simulink model "DCDC3_OL"  (R2024a)
settings: Solver=ode14x  StartTime=0.0  StopTime=0.1  FixedStep=Tstep  RelTol=1e-3
values from neighbouring files (symbols this model uses):
  D_3 = (1 - (VinNom-VdropL)/VoutNom) + deadtimesw/Tsw    (= 0.428146333333)    [DCDC_param.m]
  deadtimesw = 2.8e-6    (= 2.8e-06)    [DCDC_param.m]
  IoutNom = PCN/VoutNom    (= 1.5)    [DCDC_param.m]
  Rload = VoutNom/IoutNom    (= 33.3333333333)    [DCDC_param.m]
  RserL = 8.78e-3    (= 0.00878)    [DCDC_param.m]
  Tsw = 1/fsw    (= 0.0001)    [DCDC_param.m]    (also in adcpwm_setup.m)
  VinNom = 30    [DCDC_param.m]
  VoutNom = 50    [DCDC_param.m]
undefined symbols (not defined in the file or in its folder): den_aaf, num_aaf, Tstep
libraries: fl_lib x18, nesl_utility x17, simulink x6, spsTriangleGeneratorLib x6, ee_lib x6
settings Model: Creator=nicholas  LastModifiedBy=nicholas
settings RTWCC: GPUComputeCapability=3.5

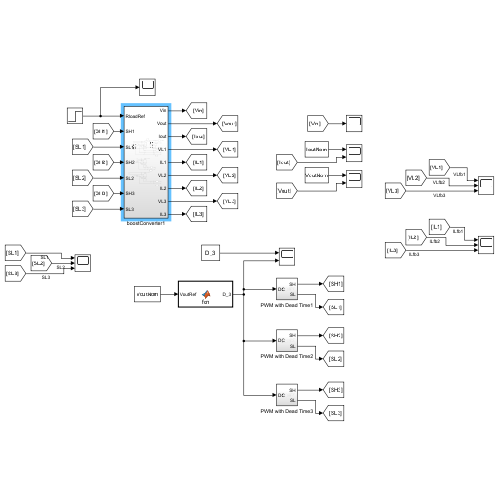
[thumbnail: Simulink's stored preview of the top-level diagram]
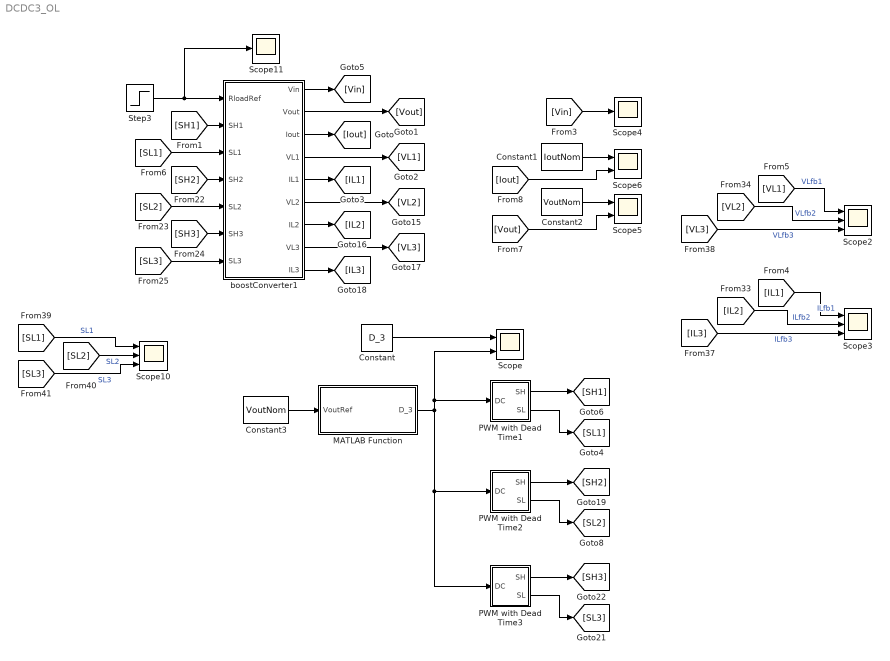
== system DCDC3_OL ==
  Constant : Constant  Value=D_3
  Constant1 : Constant  Value=IoutNom
  Constant2 : Constant  Value=VoutNom
  Constant3 : Constant  Value=VoutNom
  MATLAB Function : MATLAB Function  TreatAsAtomicUnit=on
  PWM with Dead Time1 : Subsystem
  PWM with Dead Time2 : Subsystem
  PWM with Dead Time3 : Subsystem
  Scope : Scope  NumInputPorts=2
  Scope10 : Scope  NumInputPorts=3
  Scope11 : Scope
  Scope2 : Scope  NumInputPorts=3
  Scope3 : Scope  NumInputPorts=3
  Scope4 : Scope
  Scope5 : Scope  NumInputPorts=2
  Scope6 : Scope  NumInputPorts=2
  Step3 : Step  Time=0.1  Before=Rload  After=Rload*2  SampleTime=0
  boostConverter1 : Subsystem
  wires:
  [Vin] -> Scope4/1
  [VL1] -> Scope2/1  "VLfb1"
  [IL1] -> Scope3/1  "ILfb1"
  boostConverter1/3(Iout) -> [Iout]
  boostConverter1/2(Vout) -> [Vout]
  boostConverter1/4(VL1) -> [VL1]
  boostConverter1/5(IL1) -> [IL1]
  boostConverter1/1(Vin) -> [Vin]
  [SL1] -> boostConverter1/3(SL1)
  [SH1] -> boostConverter1/2(SH1)
  Step3/1 -> Scope11/1, boostConverter1/1(RloadRef)
  boostConverter1/6(VL2) -> [VL2]
  boostConverter1/7(IL2) -> [IL2]
  boostConverter1/8(VL3) -> [VL3]
  boostConverter1/9(IL3) -> [IL3]
  [SL2] -> boostConverter1/5(SL2)
  [SH2] -> boostConverter1/4(SH2)
  [SL3] -> boostConverter1/7(SL3)
  [SH3] -> boostConverter1/6(SH3)
  [VL2] -> Scope2/2  "VLfb2"
  [VL3] -> Scope2/3  "VLfb3"
  [SL1] -> Scope10/1  "SL1"
  [SL2] -> Scope10/2  "SL2"
  [SL3] -> Scope10/3  "SL3"
  PWM with Dead Time2/1(SH) -> [SH2]
  PWM with Dead Time2/2(SL) -> [SL2]
  PWM with Dead Time1/1(SH) -> [SH1]
  PWM with Dead Time1/2(SL) -> [SL1]
  PWM with Dead Time3/1(SH) -> [SH3]
  PWM with Dead Time3/2(SL) -> [SL3]
  [IL2] -> Scope3/2  "ILfb2"
  [IL3] -> Scope3/3  "ILfb3"
  [Iout] -> Scope6/2
  [Vout] -> Scope5/2
  MATLAB Function/1(D_3) -> PWM with Dead Time1/1(DC), Scope/2, PWM with Dead Time3/1(DC), PWM with Dead Time2/1(DC)
  Constant/1 -> Scope/1
  Constant1/1 -> Scope6/1
  Constant2/1 -> Scope5/1
  Constant3/1 -> MATLAB Function/1(VoutRef)

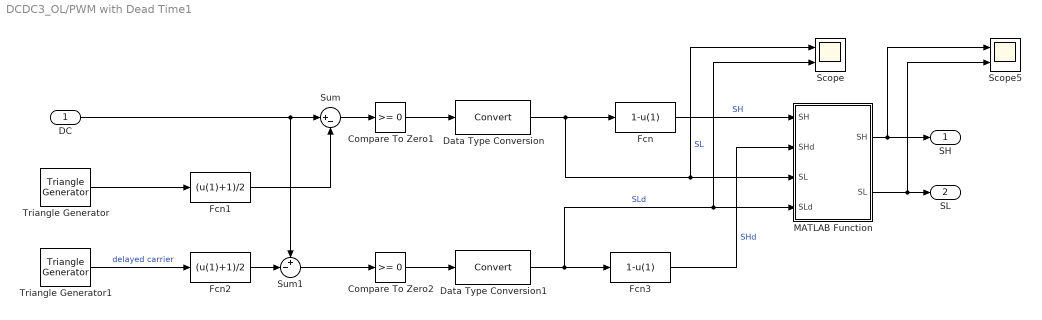
== system DCDC3_OL/PWM with Dead Time1 ==
  DC : Inport
  Compare To Zero1 : simulink/Logic and Bit Operations/Compare To Zero  relop=>=  OutDataTypeStr=boolean
  Compare To Zero2 : simulink/Logic and Bit Operations/Compare To Zero  relop=>=  OutDataTypeStr=boolean
  Data Type Conversion : DataTypeConversion  SaturateOnIntegerOverflow=off  RndMeth=Floor
  Data Type Conversion1 : DataTypeConversion  SaturateOnIntegerOverflow=off  RndMeth=Floor
  Fcn : Fcn  Expr=1-u(1)
  Fcn1 : Fcn  Expr=(u(1)+1)/2
  Fcn2 : Fcn  Expr=(u(1)+1)/2
  Fcn3 : Fcn  Expr=1-u(1)
  MATLAB Function : MATLAB Function  TreatAsAtomicUnit=on
  Scope : Scope  NumInputPorts=2
  Scope5 : Scope  NumInputPorts=2
  Sum : Sum  Inputs=|+-
  Sum1 : Sum  Inputs=+-|
  Triangle Generator : spsTriangleGeneratorLib/Triangle Generator  Freq=fsw  Phase=0  Ts=Tstep
  Triangle Generator1 : spsTriangleGeneratorLib/Triangle Generator  Freq=fsw  Phase=-(deadtimesw/Tsw)*360  Ts=Tstep
  SH : Outport
  SL : Outport  Port=2
  wires:
  Data Type Conversion/1 -> Fcn/1, Scope/1, MATLAB Function/3("SL ")  "SL"
  Fcn/1 -> MATLAB Function/1("SH ")  "SH"
  MATLAB Function/2(SL) -> SL/1, Scope5/2
  MATLAB Function/1(SH) -> SH/1, Scope5/1
  DC/1 -> Sum1/1, Sum/1
  Triangle Generator/1 -> Fcn1/1
  Sum/1 -> Compare To Zero1/1
  Fcn1/1 -> Sum/2
  Compare To Zero1/1 -> Data Type Conversion/1
  Triangle Generator1/1 -> Fcn2/1  "delayed carrier"
  Sum1/1 -> Compare To Zero2/1
  Compare To Zero2/1 -> Data Type Conversion1/1
  Fcn2/1 -> Sum1/2
  Data Type Conversion1/1 -> Fcn3/1, Scope/2, MATLAB Function/4(SLd)  "SLd"
  Fcn3/1 -> MATLAB Function/2(SHd)  "SHd"

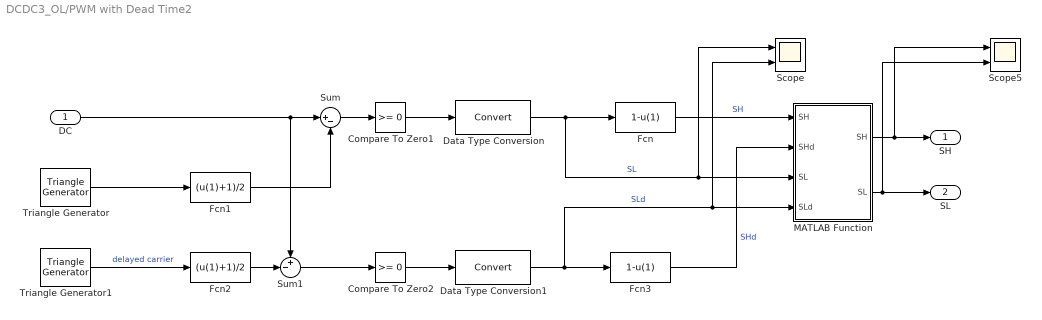
== system DCDC3_OL/PWM with Dead Time2 ==
  DC : Inport
  Compare To Zero1 : simulink/Logic and Bit Operations/Compare To Zero  relop=>=  OutDataTypeStr=boolean
  Compare To Zero2 : simulink/Logic and Bit Operations/Compare To Zero  relop=>=  OutDataTypeStr=boolean
  Data Type Conversion : DataTypeConversion  SaturateOnIntegerOverflow=off  RndMeth=Floor
  Data Type Conversion1 : DataTypeConversion  SaturateOnIntegerOverflow=off  RndMeth=Floor
  Fcn : Fcn  Expr=1-u(1)
  Fcn1 : Fcn  Expr=(u(1)+1)/2
  Fcn2 : Fcn  Expr=(u(1)+1)/2
  Fcn3 : Fcn  Expr=1-u(1)
  MATLAB Function : MATLAB Function  TreatAsAtomicUnit=on
  Scope : Scope  NumInputPorts=2
  Scope5 : Scope  NumInputPorts=2
  Sum : Sum  Inputs=|+-
  Sum1 : Sum  Inputs=+-|
  Triangle Generator : spsTriangleGeneratorLib/Triangle Generator  Freq=fsw  Phase=120  Ts=Tstep
  Triangle Generator1 : spsTriangleGeneratorLib/Triangle Generator  Freq=fsw  Phase=120-(deadtimesw/Tsw)*360  Ts=Tstep
  SH : Outport
  SL : Outport  Port=2
  wires:
  MATLAB Function/2(SL) -> SL/1, Scope5/2
  MATLAB Function/1(SH) -> SH/1, Scope5/1
  Fcn2/1 -> Sum1/2
  Compare To Zero2/1 -> Data Type Conversion1/1
  Sum1/1 -> Compare To Zero2/1
  Triangle Generator1/1 -> Fcn2/1  "delayed carrier"
  Data Type Conversion1/1 -> Scope/2, MATLAB Function/4(SLd), Fcn3/1  "SLd"
  Fcn1/1 -> Sum/2
  Sum/1 -> Compare To Zero1/1
  Triangle Generator/1 -> Fcn1/1
  DC/1 -> Sum1/1, Sum/1
  Compare To Zero1/1 -> Data Type Conversion/1
  Fcn/1 -> MATLAB Function/1("SH ")  "SH"
  Fcn3/1 -> MATLAB Function/2(SHd)  "SHd"
  Data Type Conversion/1 -> Scope/1, MATLAB Function/3("SL "), Fcn/1  "SL"

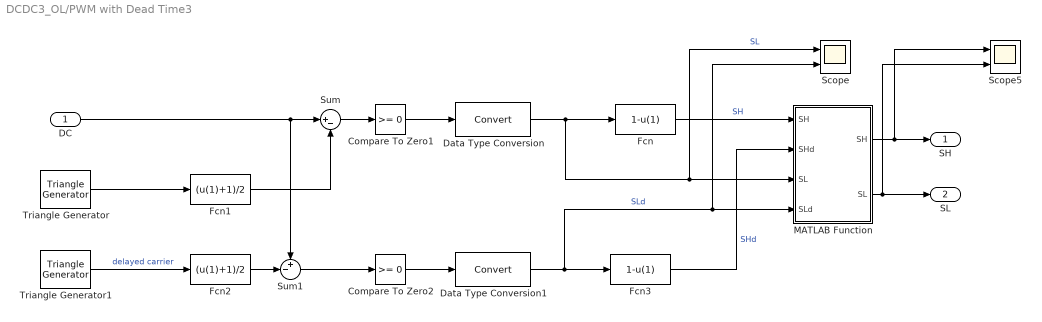
== system DCDC3_OL/PWM with Dead Time3 ==
  DC : Inport
  Compare To Zero1 : simulink/Logic and Bit Operations/Compare To Zero  relop=>=  OutDataTypeStr=boolean
  Compare To Zero2 : simulink/Logic and Bit Operations/Compare To Zero  relop=>=  OutDataTypeStr=boolean
  Data Type Conversion : DataTypeConversion  SaturateOnIntegerOverflow=off  RndMeth=Floor
  Data Type Conversion1 : DataTypeConversion  SaturateOnIntegerOverflow=off  RndMeth=Floor
  Fcn : Fcn  Expr=1-u(1)
  Fcn1 : Fcn  Expr=(u(1)+1)/2
  Fcn2 : Fcn  Expr=(u(1)+1)/2
  Fcn3 : Fcn  Expr=1-u(1)
  MATLAB Function : MATLAB Function  TreatAsAtomicUnit=on
  Scope : Scope  NumInputPorts=2
  Scope5 : Scope  NumInputPorts=2
  Sum : Sum  Inputs=|+-
  Sum1 : Sum  Inputs=+-|
  Triangle Generator : spsTriangleGeneratorLib/Triangle Generator  Freq=fsw  Phase=240  Ts=Tstep
  Triangle Generator1 : spsTriangleGeneratorLib/Triangle Generator  Freq=fsw  Phase=240-(deadtimesw/Tsw)*360  Ts=Tstep
  SH : Outport
  SL : Outport  Port=2
  wires:
  MATLAB Function/2(SL) -> SL/1, Scope5/2
  MATLAB Function/1(SH) -> SH/1, Scope5/1
  Fcn2/1 -> Sum1/2
  Compare To Zero2/1 -> Data Type Conversion1/1
  Sum1/1 -> Compare To Zero2/1
  Triangle Generator1/1 -> Fcn2/1  "delayed carrier"
  Data Type Conversion1/1 -> Scope/2, MATLAB Function/4(SLd), Fcn3/1  "SLd"
  Fcn1/1 -> Sum/2
  Sum/1 -> Compare To Zero1/1
  Triangle Generator/1 -> Fcn1/1
  DC/1 -> Sum1/1, Sum/1
  Compare To Zero1/1 -> Data Type Conversion/1
  Fcn/1 -> MATLAB Function/1("SH ")  "SH"
  Fcn3/1 -> MATLAB Function/2(SHd)  "SHd"
  Data Type Conversion/1 -> Scope/1, MATLAB Function/3("SL "), Fcn/1  "SL"

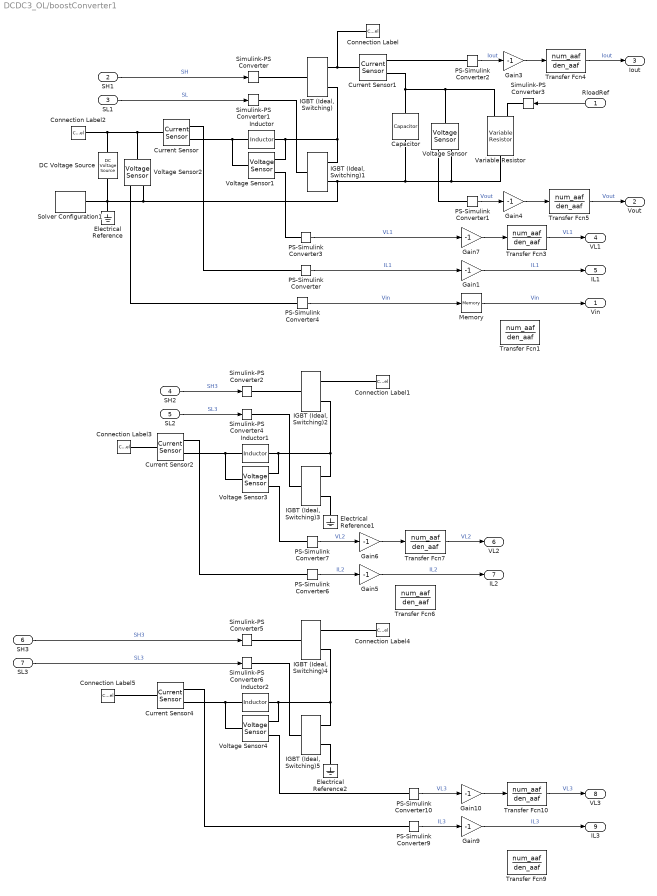
== system DCDC3_OL/boostConverter1 ==
  RloadRef : Inport
  SH1 : Inport  Port=2
  SL1 : Inport  Port=3
  SH2 : Inport  Port=4
  SL2 : Inport  Port=5
  SH3 : Inport  Port=6
  SL3 : Inport  Port=7
  Capacitor : fl_lib/Electrical/Electrical Elements/Capacitor  c=C F  r=ResrC Ohm  g=0 1/Ohm  i_specify=off  i_priority=None  i=0 A  i_nominal_specify=off  i_nominal_value=1  i_nominal_unit=A  v_specify=off  v_priority=High  v=VoutNom V  v_nominal_specify=off  v_nominal_value=1  v_nominal_unit=V  vc_specify=off  vc_priority=High  vc=0 V  vc_nominal_specify=off  vc_nominal_value=1  vc_nominal_unit=V
  Connection Label : ConnectionLabel  Label=Vout_DClink
  Connection Label1 : ConnectionLabel  Label=Vout_DClink
  Connection Label2 : ConnectionLabel  Label=Vin
  Connection Label3 : ConnectionLabel  Label=Vin
  Connection Label4 : ConnectionLabel  Label=Vout_DClink
  Connection Label5 : ConnectionLabel  Label=Vin
  Current Sensor{,1..2,4} (4 alike) : fl_lib/Electrical/Electrical Sensors/Current Sensor
  DC Voltage Source : fl_lib/Electrical/Electrical Sources/DC Voltage Source  v0=VinNom V
  Electrical Reference : fl_lib/Electrical/Electrical Elements/Electrical Reference
  Electrical Reference1 : fl_lib/Electrical/Electrical Elements/Electrical Reference
  Electrical Reference2 : fl_lib/Electrical/Electrical Elements/Electrical Reference
  Gain{1,3..7,9..10} (8 alike) : Gain  Gain=-1
  IGBT (Ideal, Switching){,1..5} (6 alike) : ee_lib/Semiconductors & Converters/IGBT (Ideal, Switching)  port_option=ee.enum.controlport.ps  Vf=0.8 V  Ron=0.001 Ohm  Goff=1e-5 1/Ohm  Vth=VthIGBT V  diode_param=ee.enum.converters.protectiondiode.nodynamics  diode_Vf=0.8 V  diode_Ron=0.001 Ohm  diode_Goff=1e-5 1/Ohm  diode_C=50e-9 F  diode_iRM=-235 A  diode_iF=300 A  diode_idot=-50 A/us  diode_trr_param=ee.enum.converters.diodeReverseParam.trr_factor  diode_trr_factor=3  diode_trr=15 us  diode_Qrr=1500 s*uA  ice_specify=off  ice_priority=None  ice=0 A  ice_nominal_specify=off  ice_nominal_value=1  ice_nominal_unit=A  vce_specify=off  vce_priority=None  vce=0 V  vce_nominal_specify=off  vce_nominal_value=1  vce_nominal_unit=V  vge_specify=off  vge_priority=None  vge=0 V  vge_nominal_specify=off  vge_nominal_value=1  vge_nominal_unit=V  thermal_loss_option=ee.enum.converters.thermalLossOption.constantvalues  Von_data=[0, .1, .6, .8, 1, 1.3, 1.6, 2, 2.4; 0, .1, .7, 1, 1.2, 1.5, 1.9, 2.4, 2.8] V  Tj=[298.15, 398.15] K  Iout_data=[0, .1, 1, 5, 10, 20, 40, 70, 100] A  Eon_data=[0, .0024, .024, .12, .2, .48, 1.04, 2.16, 3.24; 0, .003, .03, .15, .25, .6, 1.3, 2.7, 4.05] * 1e-3 J  Eoff_data=[0, .0007, .0066, .033, .066, .17, .33, .83, 1.5; 0, .001, .01, .05, .1, .25, .5, 1.2, 2.2] * 1e-3 J  Eon_data_3D=[zeros(2, 9, 3)] J  Eoff_data_3D=[zeros(2, 9, 3)] J  Tj_loss=[298.15, 398.15] K  Iout_data_loss=[0, .1, 1, 5, 10, 20, 40, 70, 100] A  tabulateWithVce=false  Vce_loss=[0, 150, 300] V  Eon_scalar=22.86e-3 J  Eoff_scalar=17.14e-3 J  Voff=300 V  Iout_scalar=600 A  useCurrentFromPreviousCycle=false  useVoltageFromPreviousCycle=false  diodeModelType=ee.enum.converters.diodeModelType.pwl  diodeTableType=ee.enum.diode.tableType.IfMat  diode_ReverseIVType=ee.enum.diode.diodeReverseIV.constant  diode_IfMat=[.07, .12, .19, 1.75, 4.24, 7.32, 11.2; .16, .3, .72, 2.14, 4.02, 6.35, 9.12] A  diode_VfMat=[.9, 1.15, 1.25, 1.5, 1.75, 2.17, 2.6, 2.85; .58, .68, .75, 1.1, 1.38, 1.77, 2.27, 2.7] V  diode_TjVec=[25, 125] degC  diode_VfVec=[.5, .7, .9, 1.3, 1.7, 2.1, 2.5] V  diode_IfVec=[.1, .2, .5, 1, 2, 4, 7, 10] A  diode_IrMat=[1e-06, 2e-06, 5e-06, 1e-05, 2.5e-05, 5e-05, .0001; 2e-06, 5e-06, 1e-05, 4e-05, 8e-05, .0002, .0005] A  diode_VrMat=[10, 100, 200, 250, 300, 325, 350; 10, 70, 160, 220, 270, 300, 320] V  diode_VrVec=[10, 20, 40, 50, 70, 80, 100] V  diode_IrVec=[1e-06, 2e-06, 5e-06, 1e-05, 2e-05, 5e-05, .0001] A  diode_Vr=-600 V  diode_Ls=150 nH  diode_Erec=0.03 J  diode_rec_loss_model=ee.enum.diode.reverseRecoveryModel.fixed  diode_ErecVal=0 J  diode_scaleWithIandV=true  diode_ErecMat=zeros(2, 3) J  diode_TjrecVec=[298.15, 398.15] K  diode_IfrecVec=[.1, 1, 10] A  diode_IrecVal=10 A  diode_VrecVal=10 V  diode_tFilter=1 / 1000 / 100 s  thermal_network_parameterization=ee.enum.thermalNetworkTopology.external  Rth=[.08, .5] K/W  Rth_Cauer=[.08, .1, .5] K/W  Rth_Foster=[.08, .14, .22, .16] K/W  thermal_mass_parameterization=ee.enum.thermalNetwork.timeconstant  thermal_mass=[.01, .5] J/K  thermal_mass_Cauer=[.01, .1, .5] J/K  thermal_mass_Foster=[.001, .005, .05, .5] J/K  thermal_time_constant=[.001, .2] s  thermal_time_constant_Cauer=[.001, .1, .2] s  thermal_time_constant_Foster=[7e-05, .0007, .01, .08] s  thermal_mass_initial_temperatures=[25, 25] degC  thermal_mass_initial_temperatures_Cauer=[25, 25, 25] degC  junction_thermal_mass=0.01 J/K  Tvec_initial_Foster=[25, 25, 25, 25] degC  no_thermal_network=0  junction_temperature_specify=off  junction_temperature_priority=None  junction_temperature=25 degC  junction_temperature_nominal_specify=off  junction_temperature_nominal_value=1  junction_temperature_nominal_unit=degC  Qj_specify=off  Qj_priority=None  Qj=0 W  Qj_nominal_specify=off  Qj_nominal_value=1  Qj_nominal_unit=W  accumulatedSwitchingLosses_specify=off  accumulatedSwitchingLosses_priority=None  accumulatedSwitchingLosses=0 J
  Inductor : fl_lib/Electrical/Electrical Elements/Inductor  l=L H  r=RserL Ohm  g=1e-9 1/Ohm  i_specify=off  i_priority=None  i=Iin A  i_nominal_specify=off  i_nominal_value=1  i_nominal_unit=A  v_specify=off  v_priority=None  v=0 V  v_nominal_specify=off  v_nominal_value=1  v_nominal_unit=V  i_L_specify=off  i_L_priority=High  i_L=0 A  i_L_nominal_specify=off  i_L_nominal_value=1  i_L_nominal_unit=A
  Inductor1 : fl_lib/Electrical/Electrical Elements/Inductor  l=L H  r=RserL Ohm  g=1e-9 1/Ohm  i_specify=off  i_priority=None  i=Iin A  i_nominal_specify=off  i_nominal_value=1  i_nominal_unit=A  v_specify=off  v_priority=None  v=0 V  v_nominal_specify=off  v_nominal_value=1  v_nominal_unit=V  i_L_specify=off  i_L_priority=High  i_L=0 A  i_L_nominal_specify=off  i_L_nominal_value=1  i_L_nominal_unit=A
  Inductor2 : fl_lib/Electrical/Electrical Elements/Inductor  l=L H  r=RserL Ohm  g=1e-9 1/Ohm  i_specify=off  i_priority=None  i=Iin A  i_nominal_specify=off  i_nominal_value=1  i_nominal_unit=A  v_specify=off  v_priority=None  v=0 V  v_nominal_specify=off  v_nominal_value=1  v_nominal_unit=V  i_L_specify=off  i_L_priority=High  i_L=0 A  i_L_nominal_specify=off  i_L_nominal_value=1  i_L_nominal_unit=A
  Memory : Memory
  PS-Simulink Converter{,1..4,6..7,9..10} (9 alike) : nesl_utility/PS-Simulink Converter  PhysicalDomain=network_engine_domain  SubClassName=ps_output  LeftPortType=input  RightPortType=output  PseudoPeriodic=off  Frequencies=[]  VectorFormat=inherit  Unit=inherit  AffineConversion=off
  Simulink-PS Converter{,1..6} (7 alike) : nesl_utility/Simulink-PS Converter  PhysicalDomain=network_engine_domain  SubClassName=ps_input  LeftPortType=input  RightPortType=output  PseudoPeriodic=off  Frequencies=[]  NoiseDistribution=none  NoiseParameters=[]  Unit=1  AffineConversion=off  FilteringAndDerivatives=provide  SimscapeFilterOrder=1  InputFilterTimeConstant=0.001  UdotUserProvided=0
  Solver Configuration1 : nesl_utility/Solver Configuration  PhysicalDomain=network_engine_domain  SubClassName=solver  LeftPortType=input  RightPortType=generic  Tones=[]  Harmonics=[]  SimulateNoise=off  Profile=off  UseLocalSampling=off  EnableSwitchedLinearOptims=on  FrequencyDomain=off  UseCCode=off  RelTol=0.001  AbsTol=1e-06  MinStep=1e-09  ToWorkspace=off  RevertToSquareIcSolve=off  NumHomotopyIterations=100  PhasorMode=off  PhasorModeNumHarmonics=1  ConsistencySolver=NEWTON_FTOL  IndexReductionMethod=DerivativeReplacement  DoDC=off  ResidualTolerance=1e-09  ConsistencyTolSource=GLOBAL  ConsistencyAbsTol=0.001  ConsistencyRelTol=0.001  ConsistencyTolFactor=0.001  UseLocalSolver=on  LocalSolverChoice=NE_TRAPEZOIDAL_ADVANCER  ResolveIndetEquations=on  FunctionEvalNumThread=1  LocalSolverSampleTime=Tstep  DoFixedCost=on  MaxNonlinIter=3  MaxModeIter=2  ComputeImpulses=off  ImpulseIterations=2  LinearAlgebra=auto  LinearAlgebraNumThread=0  EquationFormulation=NE_TIME_EF  DelaysMemoryBudget=1024  AutomaticFiltering=off  FilteringTimeConstant=0.001  PartitionStorageMethod=AS_NEEDED  PartitionMemoryBudget=1024  PartitionMethod=ROBUST  MultibodyUseLocalSolver=off  MultibodyLocalSolverChoice=ODE1  MultibodyLocalSolverSampleTime=0.001
  Transfer Fcn{1,3..7,9..10} (8 alike) : TransferFcn  Numerator=num_aaf  Denominator=den_aaf
  Variable Resistor : fl_lib/Electrical/Electrical Elements/Variable Resistor  Rmin=Rload*0.9 Ohm  thermalEnable=false  thermal_mass=1 J/K  i_specify=off  i_priority=None  i=0 A  i_nominal_specify=off  i_nominal_value=1  i_nominal_unit=A  v_specify=off  v_priority=None  v=0 V  v_nominal_specify=off  v_nominal_value=1  v_nominal_unit=V  T_specify=off  T_priority=None  T=300 K  T_nominal_specify=off  T_nominal_value=1  T_nominal_unit=K
  Voltage Sensor{,1..4} (5 alike) : fl_lib/Electrical/Electrical Sensors/Voltage Sensor
  Vin : Outport
  Vout : Outport  Port=2
  Iout : Outport  Port=3
  VL1 : Outport  Port=4
  IL1 : Outport  Port=5
  VL2 : Outport  Port=6
  IL2 : Outport  Port=7
  VL3 : Outport  Port=8
  IL3 : Outport  Port=9
  wires:
  PS-Simulink Converter4/1 -> Memory/1  "Vin"
  SH1/1 -> Simulink-PS Converter/1  "SH"
  PS-Simulink Converter2/1 -> Gain3/1  "Iout"
  PS-Simulink Converter1/1 -> Gain4/1  "Vout"
  Transfer Fcn5/1 -> Vout/1  "Vout"
  PS-Simulink Converter/1 -> Gain1/1  "IL1"
  PS-Simulink Converter3/1 -> Gain7/1  "VL1"
  SL1/1 -> Simulink-PS Converter1/1  "SL"
  Transfer Fcn3/1 -> VL1/1  "VL1"
  Gain7/1 -> Transfer Fcn3/1
  Gain1/1 -> IL1/1  "IL1"
  Memory/1 -> Vin/1  "Vin"
  Transfer Fcn4/1 -> Iout/1  "Iout"
  Gain3/1 -> Transfer Fcn4/1
  RloadRef/1 -> Simulink-PS Converter3/1
  SH2/1 -> Simulink-PS Converter2/1  "SH3"
  SL2/1 -> Simulink-PS Converter4/1  "SL3"
  PS-Simulink Converter7/1 -> Gain6/1  "VL2"
  Gain6/1 -> Transfer Fcn7/1
  Transfer Fcn7/1 -> VL2/1  "VL2"
  Gain5/1 -> IL2/1  "IL2"
  PS-Simulink Converter6/1 -> Gain5/1  "IL2"
  SL3/1 -> Simulink-PS Converter6/1  "SL3"
  PS-Simulink Converter9/1 -> Gain9/1  "IL3"
  Transfer Fcn10/1 -> VL3/1  "VL3"
  Gain9/1 -> IL3/1  "IL3"
  Gain10/1 -> Transfer Fcn10/1
  PS-Simulink Converter10/1 -> Gain10/1  "VL3"
  SH3/1 -> Simulink-PS Converter5/1  "SH3"
  Gain4/1 -> Transfer Fcn5/1
  connections:
  Current Sensor/RConn1 -- PS-Simulink Converter/LConn1
  Current Sensor/RConn2 -- Voltage Sensor1/LConn1 -- Inductor/LConn1
  Voltage Sensor2/RConn2 -- Electrical Reference/LConn1 -- Solver Configuration1/RConn1 -- DC Voltage Source/RConn1 -- "IGBT (Ideal, Switching)1"/RConn2 -- Variable Resistor/RConn1 -- Voltage Sensor/RConn2 -- Capacitor/RConn1
  PS-Simulink Converter4/LConn1 -- Voltage Sensor2/RConn1
  DC Voltage Source/LConn1 -- Voltage Sensor2/LConn1 -- Current Sensor/LConn1 -- Connection Label2/LConn1
  Current Sensor1/RConn2 -- Capacitor/LConn1 -- Variable Resistor/LConn2 -- Voltage Sensor/LConn1
  Inductor/RConn1 -- Voltage Sensor1/RConn2 -- "IGBT (Ideal, Switching)1"/RConn1 -- "IGBT (Ideal, Switching)"/RConn2
  PS-Simulink Converter3/LConn1 -- Voltage Sensor1/RConn1
  "IGBT (Ideal, Switching)"/RConn1 -- Connection Label/LConn1 -- Current Sensor1/LConn1
  "IGBT (Ideal, Switching)1"/LConn1 -- Simulink-PS Converter1/RConn1
  PS-Simulink Converter2/LConn1 -- Current Sensor1/RConn1
  PS-Simulink Converter1/LConn1 -- Voltage Sensor/RConn1
  Simulink-PS Converter/RConn1 -- "IGBT (Ideal, Switching)"/LConn1
  Variable Resistor/LConn1 -- Simulink-PS Converter3/RConn1
  "IGBT (Ideal, Switching)2"/RConn2 -- Inductor1/RConn1 -- Voltage Sensor3/RConn2 -- "IGBT (Ideal, Switching)3"/RConn1
  Inductor1/LConn1 -- Current Sensor2/RConn2 -- Voltage Sensor3/LConn1
  "IGBT (Ideal, Switching)3"/RConn2 -- Electrical Reference1/LConn1
  "IGBT (Ideal, Switching)3"/LConn1 -- Simulink-PS Converter4/RConn1
  Simulink-PS Converter2/RConn1 -- "IGBT (Ideal, Switching)2"/LConn1
  Connection Label3/LConn1 -- Current Sensor2/LConn1
  PS-Simulink Converter7/LConn1 -- Voltage Sensor3/RConn1
  PS-Simulink Converter6/LConn1 -- Current Sensor2/RConn1
  "IGBT (Ideal, Switching)4"/RConn2 -- "IGBT (Ideal, Switching)5"/RConn1 -- Inductor2/RConn1 -- Voltage Sensor4/RConn2
  Inductor2/LConn1 -- Current Sensor4/RConn2 -- Voltage Sensor4/LConn1
  "IGBT (Ideal, Switching)5"/LConn1 -- Simulink-PS Converter6/RConn1
  PS-Simulink Converter10/LConn1 -- Voltage Sensor4/RConn1
  Simulink-PS Converter5/RConn1 -- "IGBT (Ideal, Switching)4"/LConn1
  "IGBT (Ideal, Switching)5"/RConn2 -- Electrical Reference2/LConn1
  PS-Simulink Converter9/LConn1 -- Current Sensor4/RConn1
  Connection Label5/LConn1 -- Current Sensor4/LConn1
  Connection Label1/LConn1 -- "IGBT (Ideal, Switching)2"/RConn1
  Connection Label4/LConn1 -- "IGBT (Ideal, Switching)4"/RConn1

== matlab function DCDC3_OL/PWM with Dead Time2/MATLAB Function ==
  data: SH input; SHd input; SH output; SL output; SL input; SLd input
function [SH,SL] = fcn(SH,SHd,SL,SLd)

if SHd + SH > 1
    SH = 1;
else
    SH = 0;
end

if SLd + SL > 1
    SL = 1;
else
    SL = 0;
end

== matlab function DCDC3_OL/PWM with Dead Time1/MATLAB Function ==
  data: SH input; SHd input; SH output; SL output; SL input; SLd input
function [SH,SL] = fcn(SH,SHd,SL,SLd)

if SHd + SH > 1
    SH = 1;
else
    SH = 0;
end

if SLd + SL > 1
    SL = 1;
else
    SL = 0;
end

== matlab function DCDC3_OL/PWM with Dead Time3/MATLAB Function ==
  data: SH input; SHd input; SH output; SL output; SL input; SLd input
function [SH,SL] = fcn(SH,SHd,SL,SLd)

if SHd + SH > 1
    SH = 1;
else
    SH = 0;
end

if SLd + SL > 1
    SL = 1;
else
    SL = 0;
end

== matlab function DCDC3_OL/MATLAB Function ==
  data: D_3 output; VinNom parameter; RserL parameter; IoutNom parameter; VoutRef input; deadtimesw parameter; Tsw parameter
function D_3 = fcn(VinNom, RserL, IoutNom, VoutRef, deadtimesw, Tsw)

% openloop duty cycle for 1leg
D = 1 - VinNom/VoutRef;
D_3 = D/3;

%
% interleaved OL duty cycle correction
Iin = IoutNom/(1-D_3);
VdropL = Iin*RserL/3;
D_3 = (1 - (VinNom-VdropL)/VoutRef) + deadtimesw/Tsw;
%}
